simulink model "MdXX_Status"  (R2018b)
settings: Solver=FixedStepDiscrete  StartTime=0.0  StopTime=10.0  FixedStep=0.01  RelTol=1e-3
undefined symbols (not defined in the file or in its folder): data, NvStMdxxMemStatusKam_Set
libraries: RspLib x94, simulink x1
(part 1 of 2)
settings Model: Creator=sn2xws  LastModifiedBy=sn55gm
settings Model: ModifiedHistory=|
  | 25.2.19 V3.8.0 557 上到位置信号的退出，改为不再看是否有不共存的模式启动
  | 25.7.4 V3.13.0 新增Md61 Md62
settings DataIOCC: SaveFormat=StructureWithTime
settings OptimizationCC: DefaultParameterBehavior=Inlined  EnhancedBackFolding=on  PassReuseOutputArgsAs=Individual arguments  ZeroExternalMemoryAtStartup=off  ZeroInternalMemoryAtStartup=off  OptimizeBlockOrder=speed  DifferentSizesBufferReuse=on  OptimizationCustomize=off
settings DebuggingCC: ParameterTunabilityLossMsg=error
settings ModelReferenceCC: ModelReferenceNumInstancesAllowed=Single
settings SFSimCC: MATLABDynamicMemAlloc=off
settings RTWCC: SystemTargetFile=autosar.tlc  GenCodeOnly=on  TemplateMakefile=ert_default_tmf  Description=AUTOSAR  GenerateReport=on  IncludeHyperlinkInReport=on  LaunchReport=on  GenerateTraceInfo=on  GenerateTraceReport=on  GenerateTraceReportSl=on  GenerateTraceReportSf=on  GenerateTraceReportEml=on  GenerateCodeMetricsReport=on
settings CodeAppCC: ForceParamTrailComments=on  IgnoreCustomStorageClasses=off  OperatorAnnotations=on  SimulinkDataObjDesc=on  SFDataObjDesc=on  InsertBlockDesc=on
settings STFCustomTargetCC: TargetLangStandard=C99 (ISO)  MultiwordLength=256  ParMdlRefBuildCompliant=on  CompOptLevelCompliant=on  IncludeMdlTerminateFcn=off  CombineOutputUpdateFcns=on  SuppressErrorStatus=on  ERTCustomFileBanners=on  SupportNonFinite=off  SupportComplex=off  SupportContinuousTime=off  SupportNonInlinedSFcns=off  RemoveResetFunc=on  MATLABClassNameForMDSCustomization=Simulink.SoftwareTarget.ERTCustomization  AutosarCompliant=on  UseToolchainInfoCompliant=on  LookupTableObjectStructAxisOrder=2,1,3,4,...  LUTObjectStructOrderEvenSpacing=Size,Table,Breakpoints  SystemTargetFile=autosar.tlc
settings ERTTargetCC: TargetLangStandard=C99 (ISO)  ConcurrentExecutionCompliant=off  IncludeMdlTerminateFcn=off  SuppressErrorStatus=on  SupportNonFinite=off  SupportComplex=off  ModelStepFunctionPrototypeControlCompliant=off  CPPClassGenCompliant=off  AutosarCompliant=on  LookupTableObjectStructAxisOrder=2,1,3,4,...  LUTObjectStructOrderEvenSpacing=Size,Table,Breakpoints  InlinedParameterPlacement=NonHierarchical  ERTCustomFileTemplate=example_file_process.tlc  ERTFilePackagingFormat=Compact

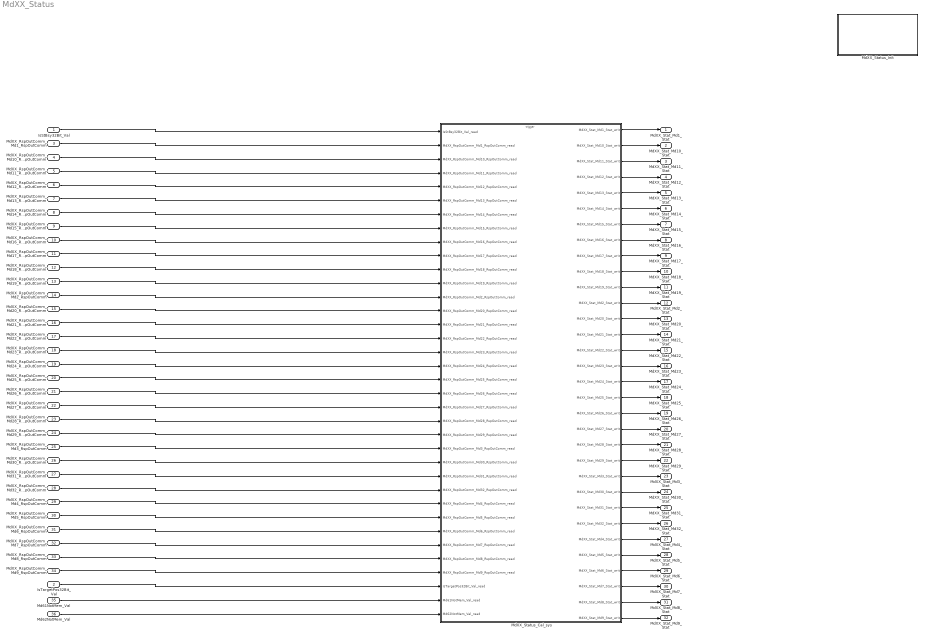
== system MdXX_Status ==
  IsStBsy32Bit_Val : Inport  OutDataTypeStr=uint32  PortDimensions=1
  IsTargetPos32Bit_Val : Inport  Port=2  OutDataTypeStr=uint32  PortDimensions=1
  MdXX_RspOutComm_Md1_RspOutComm : Inport  Port=3  OutDataTypeStr=uint8  PortDimensions=1
  MdXX_RspOutComm_Md10_RspOutComm : Inport  Port=4  OutDataTypeStr=uint8  PortDimensions=1
  MdXX_RspOutComm_Md11_RspOutComm : Inport  Port=5  OutDataTypeStr=uint8  PortDimensions=1
  MdXX_RspOutComm_Md12_RspOutComm : Inport  Port=6  OutDataTypeStr=uint8  PortDimensions=1
  MdXX_RspOutComm_Md13_RspOutComm : Inport  Port=7  OutDataTypeStr=uint8  PortDimensions=1
  MdXX_RspOutComm_Md14_RspOutComm : Inport  Port=8  OutDataTypeStr=uint8  PortDimensions=1
  MdXX_RspOutComm_Md15_RspOutComm : Inport  Port=9  OutDataTypeStr=uint8  PortDimensions=1
  MdXX_RspOutComm_Md16_RspOutComm : Inport  Port=10  OutDataTypeStr=uint8  PortDimensions=1
  MdXX_RspOutComm_Md17_RspOutComm : Inport  Port=11  OutDataTypeStr=uint8  PortDimensions=1
  MdXX_RspOutComm_Md18_RspOutComm : Inport  Port=12  OutDataTypeStr=uint8  PortDimensions=1
  MdXX_RspOutComm_Md19_RspOutComm : Inport  Port=13  OutDataTypeStr=uint8  PortDimensions=1
  MdXX_RspOutComm_Md2_RspOutComm : Inport  Port=14  OutDataTypeStr=uint8  PortDimensions=1
  MdXX_RspOutComm_Md20_RspOutComm : Inport  Port=15  OutDataTypeStr=uint8  PortDimensions=1
  MdXX_RspOutComm_Md21_RspOutComm : Inport  Port=16  OutDataTypeStr=uint8  PortDimensions=1
  MdXX_RspOutComm_Md22_RspOutComm : Inport  Port=17  OutDataTypeStr=uint8  PortDimensions=1
  MdXX_RspOutComm_Md23_RspOutComm : Inport  Port=18  OutDataTypeStr=uint8  PortDimensions=1
  MdXX_RspOutComm_Md24_RspOutComm : Inport  Port=19  OutDataTypeStr=uint8  PortDimensions=1
  MdXX_RspOutComm_Md25_RspOutComm : Inport  Port=20  OutDataTypeStr=uint8  PortDimensions=1
  MdXX_RspOutComm_Md26_RspOutComm : Inport  Port=21  OutDataTypeStr=uint8  PortDimensions=1
  MdXX_RspOutComm_Md27_RspOutComm : Inport  Port=22  OutDataTypeStr=uint8  PortDimensions=1
  MdXX_RspOutComm_Md28_RspOutComm : Inport  Port=23  OutDataTypeStr=uint8  PortDimensions=1
  MdXX_RspOutComm_Md29_RspOutComm : Inport  Port=24  OutDataTypeStr=uint8  PortDimensions=1
  MdXX_RspOutComm_Md3_RspOutComm : Inport  Port=25  OutDataTypeStr=uint8  PortDimensions=1
  MdXX_RspOutComm_Md30_RspOutComm : Inport  Port=26  OutDataTypeStr=uint8  PortDimensions=1
  MdXX_RspOutComm_Md31_RspOutComm : Inport  Port=27  OutDataTypeStr=uint8  PortDimensions=1
  MdXX_RspOutComm_Md32_RspOutComm : Inport  Port=28  OutDataTypeStr=uint8  PortDimensions=1
  MdXX_RspOutComm_Md4_RspOutComm : Inport  Port=29  OutDataTypeStr=uint8  PortDimensions=1
  MdXX_RspOutComm_Md5_RspOutComm : Inport  Port=30  OutDataTypeStr=uint8  PortDimensions=1
  MdXX_RspOutComm_Md6_RspOutComm : Inport  Port=31  OutDataTypeStr=uint8  PortDimensions=1
  MdXX_RspOutComm_Md7_RspOutComm : Inport  Port=32  OutDataTypeStr=uint8  PortDimensions=1
  MdXX_RspOutComm_Md8_RspOutComm : Inport  Port=33  OutDataTypeStr=uint8  PortDimensions=1
  MdXX_RspOutComm_Md9_RspOutComm : Inport  Port=34  OutDataTypeStr=uint8  PortDimensions=1
  Md61NotMem_Val : Inport  Port=35  OutDataTypeStr=boolean  PortDimensions=1
  Md62NotMem_Val : Inport  Port=36  OutDataTypeStr=boolean  PortDimensions=1
  MdXX_Status_Cal_sys : Subsystem
  MdXX_Status_Init : Subsystem
  MdXX_Stat_Md1_Stat : Outport  OutDataTypeStr=uint8  PortDimensions=1
  MdXX_Stat_Md10_Stat : Outport  Port=2  OutDataTypeStr=uint8  PortDimensions=1
  MdXX_Stat_Md11_Stat : Outport  Port=3  OutDataTypeStr=uint8  PortDimensions=1
  MdXX_Stat_Md12_Stat : Outport  Port=4  OutDataTypeStr=uint8  PortDimensions=1
  MdXX_Stat_Md13_Stat : Outport  Port=5  OutDataTypeStr=uint8  PortDimensions=1
  MdXX_Stat_Md14_Stat : Outport  Port=6  OutDataTypeStr=uint8  PortDimensions=1
  MdXX_Stat_Md15_Stat : Outport  Port=7  OutDataTypeStr=uint8  PortDimensions=1
  MdXX_Stat_Md16_Stat : Outport  Port=8  OutDataTypeStr=uint8  PortDimensions=1
  MdXX_Stat_Md17_Stat : Outport  Port=9  OutDataTypeStr=uint8  PortDimensions=1
  MdXX_Stat_Md18_Stat : Outport  Port=10  OutDataTypeStr=uint8  PortDimensions=1
  MdXX_Stat_Md19_Stat : Outport  Port=11  OutDataTypeStr=uint8  PortDimensions=1
  MdXX_Stat_Md2_Stat : Outport  Port=12  OutDataTypeStr=uint8  PortDimensions=1
  MdXX_Stat_Md20_Stat : Outport  Port=13  OutDataTypeStr=uint8  PortDimensions=1
  MdXX_Stat_Md21_Stat : Outport  Port=14  OutDataTypeStr=uint8  PortDimensions=1
  MdXX_Stat_Md22_Stat : Outport  Port=15  OutDataTypeStr=uint8  PortDimensions=1
  MdXX_Stat_Md23_Stat : Outport  Port=16  OutDataTypeStr=uint8  PortDimensions=1
  MdXX_Stat_Md24_Stat : Outport  Port=17  OutDataTypeStr=uint8  PortDimensions=1
  MdXX_Stat_Md25_Stat : Outport  Port=18  OutDataTypeStr=uint8  PortDimensions=1
  MdXX_Stat_Md26_Stat : Outport  Port=19  OutDataTypeStr=uint8  PortDimensions=1
  MdXX_Stat_Md27_Stat : Outport  Port=20  OutDataTypeStr=uint8  PortDimensions=1
  MdXX_Stat_Md28_Stat : Outport  Port=21  OutDataTypeStr=uint8  PortDimensions=1
  MdXX_Stat_Md29_Stat : Outport  Port=22  OutDataTypeStr=uint8  PortDimensions=1
  MdXX_Stat_Md3_Stat : Outport  Port=23  OutDataTypeStr=uint8  PortDimensions=1
  MdXX_Stat_Md30_Stat : Outport  Port=24  OutDataTypeStr=uint8  PortDimensions=1
  MdXX_Stat_Md31_Stat : Outport  Port=25  OutDataTypeStr=uint8  PortDimensions=1
  MdXX_Stat_Md32_Stat : Outport  Port=26  OutDataTypeStr=uint8  PortDimensions=1
  MdXX_Stat_Md4_Stat : Outport  Port=27  OutDataTypeStr=uint8  PortDimensions=1
  MdXX_Stat_Md5_Stat : Outport  Port=28  OutDataTypeStr=uint8  PortDimensions=1
  MdXX_Stat_Md6_Stat : Outport  Port=29  OutDataTypeStr=uint8  PortDimensions=1
  MdXX_Stat_Md7_Stat : Outport  Port=30  OutDataTypeStr=uint8  PortDimensions=1
  MdXX_Stat_Md8_Stat : Outport  Port=31  OutDataTypeStr=uint8  PortDimensions=1
  MdXX_Stat_Md9_Stat : Outport  Port=32  OutDataTypeStr=uint8  PortDimensions=1
  wires:
  IsStBsy32Bit_Val/1 -> MdXX_Status_Cal_sys/1(IsStBsy32Bit_Val_read)
  IsTargetPos32Bit_Val/1 -> MdXX_Status_Cal_sys/34(IsTargetPos32Bit_Val_read)
  MdXX_RspOutComm_Md1_RspOutComm/1 -> MdXX_Status_Cal_sys/2(MdXX_RspOutComm_Md1_RspOutComm_read)
  MdXX_RspOutComm_Md10_RspOutComm/1 -> MdXX_Status_Cal_sys/3(MdXX_RspOutComm_Md10_RspOutComm_read)
  MdXX_RspOutComm_Md11_RspOutComm/1 -> MdXX_Status_Cal_sys/4(MdXX_RspOutComm_Md11_RspOutComm_read)
  MdXX_RspOutComm_Md12_RspOutComm/1 -> MdXX_Status_Cal_sys/5(MdXX_RspOutComm_Md12_RspOutComm_read)
  MdXX_RspOutComm_Md13_RspOutComm/1 -> MdXX_Status_Cal_sys/6(MdXX_RspOutComm_Md13_RspOutComm_read)
  MdXX_RspOutComm_Md14_RspOutComm/1 -> MdXX_Status_Cal_sys/7(MdXX_RspOutComm_Md14_RspOutComm_read)
  MdXX_RspOutComm_Md15_RspOutComm/1 -> MdXX_Status_Cal_sys/8(MdXX_RspOutComm_Md15_RspOutComm_read)
  MdXX_RspOutComm_Md16_RspOutComm/1 -> MdXX_Status_Cal_sys/9(MdXX_RspOutComm_Md16_RspOutComm_read)
  MdXX_RspOutComm_Md17_RspOutComm/1 -> MdXX_Status_Cal_sys/10(MdXX_RspOutComm_Md17_RspOutComm_read)
  MdXX_RspOutComm_Md18_RspOutComm/1 -> MdXX_Status_Cal_sys/11(MdXX_RspOutComm_Md18_RspOutComm_read)
  MdXX_RspOutComm_Md19_RspOutComm/1 -> MdXX_Status_Cal_sys/12(MdXX_RspOutComm_Md19_RspOutComm_read)
  MdXX_RspOutComm_Md2_RspOutComm/1 -> MdXX_Status_Cal_sys/13(MdXX_RspOutComm_Md2_RspOutComm_read)
  MdXX_RspOutComm_Md20_RspOutComm/1 -> MdXX_Status_Cal_sys/14(MdXX_RspOutComm_Md20_RspOutComm_read)
  MdXX_RspOutComm_Md21_RspOutComm/1 -> MdXX_Status_Cal_sys/15(MdXX_RspOutComm_Md21_RspOutComm_read)
  MdXX_RspOutComm_Md22_RspOutComm/1 -> MdXX_Status_Cal_sys/16(MdXX_RspOutComm_Md22_RspOutComm_read)
  MdXX_RspOutComm_Md23_RspOutComm/1 -> MdXX_Status_Cal_sys/17(MdXX_RspOutComm_Md23_RspOutComm_read)
  MdXX_RspOutComm_Md24_RspOutComm/1 -> MdXX_Status_Cal_sys/18(MdXX_RspOutComm_Md24_RspOutComm_read)
  MdXX_RspOutComm_Md25_RspOutComm/1 -> MdXX_Status_Cal_sys/19(MdXX_RspOutComm_Md25_RspOutComm_read)
  MdXX_RspOutComm_Md26_RspOutComm/1 -> MdXX_Status_Cal_sys/20(MdXX_RspOutComm_Md26_RspOutComm_read)
  MdXX_RspOutComm_Md27_RspOutComm/1 -> MdXX_Status_Cal_sys/21(MdXX_RspOutComm_Md27_RspOutComm_read)
  MdXX_RspOutComm_Md28_RspOutComm/1 -> MdXX_Status_Cal_sys/22(MdXX_RspOutComm_Md28_RspOutComm_read)
  MdXX_RspOutComm_Md29_RspOutComm/1 -> MdXX_Status_Cal_sys/23(MdXX_RspOutComm_Md29_RspOutComm_read)
  MdXX_RspOutComm_Md3_RspOutComm/1 -> MdXX_Status_Cal_sys/24(MdXX_RspOutComm_Md3_RspOutComm_read)
  MdXX_RspOutComm_Md30_RspOutComm/1 -> MdXX_Status_Cal_sys/25(MdXX_RspOutComm_Md30_RspOutComm_read)
  MdXX_RspOutComm_Md31_RspOutComm/1 -> MdXX_Status_Cal_sys/26(MdXX_RspOutComm_Md31_RspOutComm_read)
  MdXX_RspOutComm_Md32_RspOutComm/1 -> MdXX_Status_Cal_sys/27(MdXX_RspOutComm_Md32_RspOutComm_read)
  MdXX_RspOutComm_Md4_RspOutComm/1 -> MdXX_Status_Cal_sys/28(MdXX_RspOutComm_Md4_RspOutComm_read)
  MdXX_RspOutComm_Md5_RspOutComm/1 -> MdXX_Status_Cal_sys/29(MdXX_RspOutComm_Md5_RspOutComm_read)
  MdXX_RspOutComm_Md6_RspOutComm/1 -> MdXX_Status_Cal_sys/30(MdXX_RspOutComm_Md6_RspOutComm_read)
  MdXX_RspOutComm_Md7_RspOutComm/1 -> MdXX_Status_Cal_sys/31(MdXX_RspOutComm_Md7_RspOutComm_read)
  MdXX_RspOutComm_Md8_RspOutComm/1 -> MdXX_Status_Cal_sys/32(MdXX_RspOutComm_Md8_RspOutComm_read)
  MdXX_RspOutComm_Md9_RspOutComm/1 -> MdXX_Status_Cal_sys/33(MdXX_RspOutComm_Md9_RspOutComm_read)
  MdXX_Status_Cal_sys/1(MdXX_Stat_Md1_Stat_write) -> MdXX_Stat_Md1_Stat/1
  MdXX_Status_Cal_sys/2(MdXX_Stat_Md10_Stat_write) -> MdXX_Stat_Md10_Stat/1
  MdXX_Status_Cal_sys/3(MdXX_Stat_Md11_Stat_write) -> MdXX_Stat_Md11_Stat/1
  MdXX_Status_Cal_sys/4(MdXX_Stat_Md12_Stat_write) -> MdXX_Stat_Md12_Stat/1
  MdXX_Status_Cal_sys/5(MdXX_Stat_Md13_Stat_write) -> MdXX_Stat_Md13_Stat/1
  MdXX_Status_Cal_sys/6(MdXX_Stat_Md14_Stat_write) -> MdXX_Stat_Md14_Stat/1
  MdXX_Status_Cal_sys/7(MdXX_Stat_Md15_Stat_write) -> MdXX_Stat_Md15_Stat/1
  MdXX_Status_Cal_sys/8(MdXX_Stat_Md16_Stat_write) -> MdXX_Stat_Md16_Stat/1
  MdXX_Status_Cal_sys/9(MdXX_Stat_Md17_Stat_write) -> MdXX_Stat_Md17_Stat/1
  MdXX_Status_Cal_sys/10(MdXX_Stat_Md18_Stat_write) -> MdXX_Stat_Md18_Stat/1
  MdXX_Status_Cal_sys/11(MdXX_Stat_Md19_Stat_write) -> MdXX_Stat_Md19_Stat/1
  MdXX_Status_Cal_sys/12(MdXX_Stat_Md2_Stat_write) -> MdXX_Stat_Md2_Stat/1
  MdXX_Status_Cal_sys/13(MdXX_Stat_Md20_Stat_write) -> MdXX_Stat_Md20_Stat/1
  MdXX_Status_Cal_sys/14(MdXX_Stat_Md21_Stat_write) -> MdXX_Stat_Md21_Stat/1
  MdXX_Status_Cal_sys/15(MdXX_Stat_Md22_Stat_write) -> MdXX_Stat_Md22_Stat/1
  MdXX_Status_Cal_sys/16(MdXX_Stat_Md23_Stat_write) -> MdXX_Stat_Md23_Stat/1
  MdXX_Status_Cal_sys/17(MdXX_Stat_Md24_Stat_write) -> MdXX_Stat_Md24_Stat/1
  MdXX_Status_Cal_sys/18(MdXX_Stat_Md25_Stat_write) -> MdXX_Stat_Md25_Stat/1
  MdXX_Status_Cal_sys/19(MdXX_Stat_Md26_Stat_write) -> MdXX_Stat_Md26_Stat/1
  MdXX_Status_Cal_sys/20(MdXX_Stat_Md27_Stat_write) -> MdXX_Stat_Md27_Stat/1
  MdXX_Status_Cal_sys/21(MdXX_Stat_Md28_Stat_write) -> MdXX_Stat_Md28_Stat/1
  MdXX_Status_Cal_sys/22(MdXX_Stat_Md29_Stat_write) -> MdXX_Stat_Md29_Stat/1
  MdXX_Status_Cal_sys/23(MdXX_Stat_Md3_Stat_write) -> MdXX_Stat_Md3_Stat/1
  MdXX_Status_Cal_sys/24(MdXX_Stat_Md30_Stat_write) -> MdXX_Stat_Md30_Stat/1
  MdXX_Status_Cal_sys/25(MdXX_Stat_Md31_Stat_write) -> MdXX_Stat_Md31_Stat/1
  MdXX_Status_Cal_sys/26(MdXX_Stat_Md32_Stat_write) -> MdXX_Stat_Md32_Stat/1
  MdXX_Status_Cal_sys/27(MdXX_Stat_Md4_Stat_write) -> MdXX_Stat_Md4_Stat/1
  MdXX_Status_Cal_sys/28(MdXX_Stat_Md5_Stat_write) -> MdXX_Stat_Md5_Stat/1
  MdXX_Status_Cal_sys/29(MdXX_Stat_Md6_Stat_write) -> MdXX_Stat_Md6_Stat/1
  MdXX_Status_Cal_sys/30(MdXX_Stat_Md7_Stat_write) -> MdXX_Stat_Md7_Stat/1
  MdXX_Status_Cal_sys/31(MdXX_Stat_Md8_Stat_write) -> MdXX_Stat_Md8_Stat/1
  MdXX_Status_Cal_sys/32(MdXX_Stat_Md9_Stat_write) -> MdXX_Stat_Md9_Stat/1
  Md61NotMem_Val/1 -> MdXX_Status_Cal_sys/35(Md61NotMem_Val_read)
  Md62NotMem_Val/1 -> MdXX_Status_Cal_sys/36(Md62NotMem_Val_read)

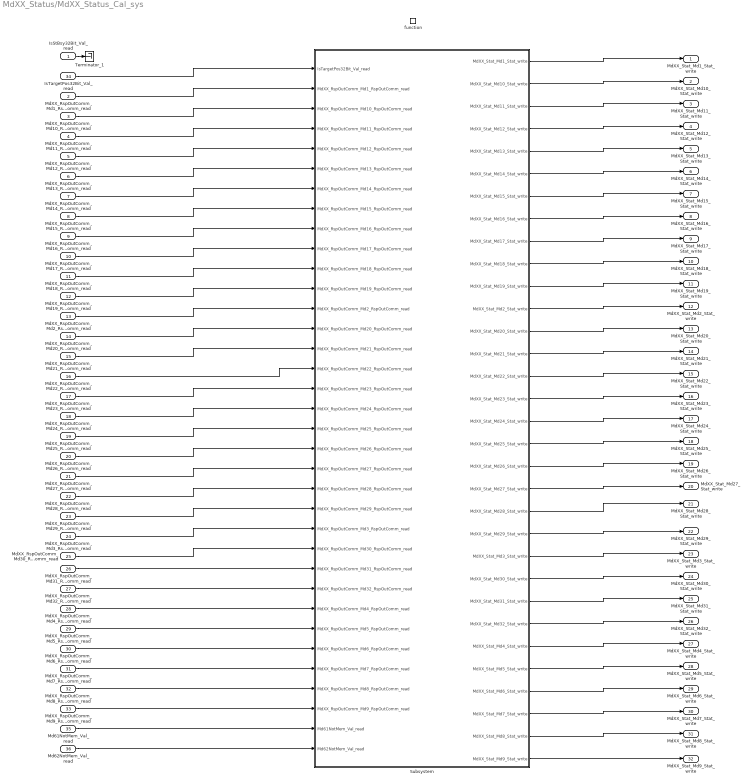
== system MdXX_Status/MdXX_Status_Cal_sys ==
  IsStBsy32Bit_Val_read : Inport
  MdXX_RspOutComm_Md1_RspOutComm_read : Inport  Port=2
  MdXX_RspOutComm_Md10_RspOutComm_read : Inport  Port=3
  MdXX_RspOutComm_Md11_RspOutComm_read : Inport  Port=4
  MdXX_RspOutComm_Md12_RspOutComm_read : Inport  Port=5
  MdXX_RspOutComm_Md13_RspOutComm_read : Inport  Port=6
  MdXX_RspOutComm_Md14_RspOutComm_read : Inport  Port=7
  MdXX_RspOutComm_Md15_RspOutComm_read : Inport  Port=8
  MdXX_RspOutComm_Md16_RspOutComm_read : Inport  Port=9
  MdXX_RspOutComm_Md17_RspOutComm_read : Inport  Port=10
  MdXX_RspOutComm_Md18_RspOutComm_read : Inport  Port=11
  MdXX_RspOutComm_Md19_RspOutComm_read : Inport  Port=12
  MdXX_RspOutComm_Md2_RspOutComm_read : Inport  Port=13
  MdXX_RspOutComm_Md20_RspOutComm_read : Inport  Port=14
  MdXX_RspOutComm_Md21_RspOutComm_read : Inport  Port=15
  MdXX_RspOutComm_Md22_RspOutComm_read : Inport  Port=16
  MdXX_RspOutComm_Md23_RspOutComm_read : Inport  Port=17
  MdXX_RspOutComm_Md24_RspOutComm_read : Inport  Port=18
  MdXX_RspOutComm_Md25_RspOutComm_read : Inport  Port=19
  MdXX_RspOutComm_Md26_RspOutComm_read : Inport  Port=20
  MdXX_RspOutComm_Md27_RspOutComm_read : Inport  Port=21
  MdXX_RspOutComm_Md28_RspOutComm_read : Inport  Port=22
  MdXX_RspOutComm_Md29_RspOutComm_read : Inport  Port=23
  MdXX_RspOutComm_Md3_RspOutComm_read : Inport  Port=24
  MdXX_RspOutComm_Md30_RspOutComm_read : Inport  Port=25
  MdXX_RspOutComm_Md31_RspOutComm_read : Inport  Port=26
  MdXX_RspOutComm_Md32_RspOutComm_read : Inport  Port=27
  MdXX_RspOutComm_Md4_RspOutComm_read : Inport  Port=28
  MdXX_RspOutComm_Md5_RspOutComm_read : Inport  Port=29
  MdXX_RspOutComm_Md6_RspOutComm_read : Inport  Port=30
  MdXX_RspOutComm_Md7_RspOutComm_read : Inport  Port=31
  MdXX_RspOutComm_Md8_RspOutComm_read : Inport  Port=32
  MdXX_RspOutComm_Md9_RspOutComm_read : Inport  Port=33
  IsTargetPos32Bit_Val_read : Inport  Port=34
  Md61NotMem_Val_read : Inport  Port=35
  Md62NotMem_Val_read : Inport  Port=36
  function : TriggerPort  TriggerType=function-call  IsSimulinkFunction=on  FunctionName=MdXX_Status_Cal  VariantControl=(inherit)
  Subsystem : Subsystem
  Terminator_1 : Terminator
  MdXX_Stat_Md1_Stat_write : Outport  InitialOutput=0
  MdXX_Stat_Md10_Stat_write : Outport  Port=2  InitialOutput=0
  MdXX_Stat_Md11_Stat_write : Outport  Port=3  InitialOutput=0
  MdXX_Stat_Md12_Stat_write : Outport  Port=4  InitialOutput=0
  MdXX_Stat_Md13_Stat_write : Outport  Port=5  InitialOutput=0
  MdXX_Stat_Md14_Stat_write : Outport  Port=6  InitialOutput=0
  MdXX_Stat_Md15_Stat_write : Outport  Port=7  InitialOutput=0
  MdXX_Stat_Md16_Stat_write : Outport  Port=8  InitialOutput=0
  MdXX_Stat_Md17_Stat_write : Outport  Port=9  InitialOutput=0
  MdXX_Stat_Md18_Stat_write : Outport  Port=10  InitialOutput=0
  MdXX_Stat_Md19_Stat_write : Outport  Port=11  InitialOutput=0
  MdXX_Stat_Md2_Stat_write : Outport  Port=12  InitialOutput=0
  MdXX_Stat_Md20_Stat_write : Outport  Port=13  InitialOutput=0
  MdXX_Stat_Md21_Stat_write : Outport  Port=14  InitialOutput=0
  MdXX_Stat_Md22_Stat_write : Outport  Port=15  InitialOutput=0
  MdXX_Stat_Md23_Stat_write : Outport  Port=16  InitialOutput=0
  MdXX_Stat_Md24_Stat_write : Outport  Port=17  InitialOutput=0
  MdXX_Stat_Md25_Stat_write : Outport  Port=18  InitialOutput=0
  MdXX_Stat_Md26_Stat_write : Outport  Port=19  InitialOutput=0
  MdXX_Stat_Md27_Stat_write : Outport  Port=20  InitialOutput=0
  MdXX_Stat_Md28_Stat_write : Outport  Port=21  InitialOutput=0
  MdXX_Stat_Md29_Stat_write : Outport  Port=22  InitialOutput=0
  MdXX_Stat_Md3_Stat_write : Outport  Port=23  InitialOutput=0
  MdXX_Stat_Md30_Stat_write : Outport  Port=24  InitialOutput=0
  MdXX_Stat_Md31_Stat_write : Outport  Port=25  InitialOutput=0
  MdXX_Stat_Md32_Stat_write : Outport  Port=26  InitialOutput=0
  MdXX_Stat_Md4_Stat_write : Outport  Port=27  InitialOutput=0
  MdXX_Stat_Md5_Stat_write : Outport  Port=28  InitialOutput=0
  MdXX_Stat_Md6_Stat_write : Outport  Port=29  InitialOutput=0
  MdXX_Stat_Md7_Stat_write : Outport  Port=30  InitialOutput=0
  MdXX_Stat_Md8_Stat_write : Outport  Port=31  InitialOutput=0
  MdXX_Stat_Md9_Stat_write : Outport  Port=32  InitialOutput=0
  wires:
  Subsystem/1(MdXX_Stat_Md1_Stat_write) -> MdXX_Stat_Md1_Stat_write/1
  Subsystem/2(MdXX_Stat_Md10_Stat_write) -> MdXX_Stat_Md10_Stat_write/1
  Subsystem/3(MdXX_Stat_Md11_Stat_write) -> MdXX_Stat_Md11_Stat_write/1
  Subsystem/4(MdXX_Stat_Md12_Stat_write) -> MdXX_Stat_Md12_Stat_write/1
  Subsystem/5(MdXX_Stat_Md13_Stat_write) -> MdXX_Stat_Md13_Stat_write/1
  Subsystem/6(MdXX_Stat_Md14_Stat_write) -> MdXX_Stat_Md14_Stat_write/1
  Subsystem/7(MdXX_Stat_Md15_Stat_write) -> MdXX_Stat_Md15_Stat_write/1
  Subsystem/8(MdXX_Stat_Md16_Stat_write) -> MdXX_Stat_Md16_Stat_write/1
  Subsystem/9(MdXX_Stat_Md17_Stat_write) -> MdXX_Stat_Md17_Stat_write/1
  Subsystem/10(MdXX_Stat_Md18_Stat_write) -> MdXX_Stat_Md18_Stat_write/1
  Subsystem/11(MdXX_Stat_Md19_Stat_write) -> MdXX_Stat_Md19_Stat_write/1
  Subsystem/12(MdXX_Stat_Md2_Stat_write) -> MdXX_Stat_Md2_Stat_write/1
  Subsystem/13(MdXX_Stat_Md20_Stat_write) -> MdXX_Stat_Md20_Stat_write/1
  Subsystem/14(MdXX_Stat_Md21_Stat_write) -> MdXX_Stat_Md21_Stat_write/1
  Subsystem/15(MdXX_Stat_Md22_Stat_write) -> MdXX_Stat_Md22_Stat_write/1
  Subsystem/16(MdXX_Stat_Md23_Stat_write) -> MdXX_Stat_Md23_Stat_write/1
  Subsystem/17(MdXX_Stat_Md24_Stat_write) -> MdXX_Stat_Md24_Stat_write/1
  Subsystem/18(MdXX_Stat_Md25_Stat_write) -> MdXX_Stat_Md25_Stat_write/1
  Subsystem/19(MdXX_Stat_Md26_Stat_write) -> MdXX_Stat_Md26_Stat_write/1
  Subsystem/20(MdXX_Stat_Md27_Stat_write) -> MdXX_Stat_Md27_Stat_write/1
  Subsystem/21(MdXX_Stat_Md28_Stat_write) -> MdXX_Stat_Md28_Stat_write/1
  Subsystem/22(MdXX_Stat_Md29_Stat_write) -> MdXX_Stat_Md29_Stat_write/1
  Subsystem/23(MdXX_Stat_Md3_Stat_write) -> MdXX_Stat_Md3_Stat_write/1
  Subsystem/24(MdXX_Stat_Md30_Stat_write) -> MdXX_Stat_Md30_Stat_write/1
  Subsystem/25(MdXX_Stat_Md31_Stat_write) -> MdXX_Stat_Md31_Stat_write/1
  Subsystem/26(MdXX_Stat_Md32_Stat_write) -> MdXX_Stat_Md32_Stat_write/1
  Subsystem/27(MdXX_Stat_Md4_Stat_write) -> MdXX_Stat_Md4_Stat_write/1
  Subsystem/28(MdXX_Stat_Md5_Stat_write) -> MdXX_Stat_Md5_Stat_write/1
  Subsystem/29(MdXX_Stat_Md6_Stat_write) -> MdXX_Stat_Md6_Stat_write/1
  Subsystem/30(MdXX_Stat_Md7_Stat_write) -> MdXX_Stat_Md7_Stat_write/1
  Subsystem/31(MdXX_Stat_Md8_Stat_write) -> MdXX_Stat_Md8_Stat_write/1
  Subsystem/32(MdXX_Stat_Md9_Stat_write) -> MdXX_Stat_Md9_Stat_write/1
  IsTargetPos32Bit_Val_read/1 -> Subsystem/1(IsTargetPos32Bit_Val_read)
  MdXX_RspOutComm_Md1_RspOutComm_read/1 -> Subsystem/2(MdXX_RspOutComm_Md1_RspOutComm_read)
  MdXX_RspOutComm_Md10_RspOutComm_read/1 -> Subsystem/3(MdXX_RspOutComm_Md10_RspOutComm_read)
  MdXX_RspOutComm_Md11_RspOutComm_read/1 -> Subsystem/4(MdXX_RspOutComm_Md11_RspOutComm_read)
  MdXX_RspOutComm_Md12_RspOutComm_read/1 -> Subsystem/5(MdXX_RspOutComm_Md12_RspOutComm_read)
  MdXX_RspOutComm_Md13_RspOutComm_read/1 -> Subsystem/6(MdXX_RspOutComm_Md13_RspOutComm_read)
  MdXX_RspOutComm_Md14_RspOutComm_read/1 -> Subsystem/7(MdXX_RspOutComm_Md14_RspOutComm_read)
  MdXX_RspOutComm_Md15_RspOutComm_read/1 -> Subsystem/8(MdXX_RspOutComm_Md15_RspOutComm_read)
  MdXX_RspOutComm_Md16_RspOutComm_read/1 -> Subsystem/9(MdXX_RspOutComm_Md16_RspOutComm_read)
  MdXX_RspOutComm_Md17_RspOutComm_read/1 -> Subsystem/10(MdXX_RspOutComm_Md17_RspOutComm_read)
  MdXX_RspOutComm_Md18_RspOutComm_read/1 -> Subsystem/11(MdXX_RspOutComm_Md18_RspOutComm_read)
  MdXX_RspOutComm_Md19_RspOutComm_read/1 -> Subsystem/12(MdXX_RspOutComm_Md19_RspOutComm_read)
  MdXX_RspOutComm_Md2_RspOutComm_read/1 -> Subsystem/13(MdXX_RspOutComm_Md2_RspOutComm_read)
  MdXX_RspOutComm_Md20_RspOutComm_read/1 -> Subsystem/14(MdXX_RspOutComm_Md20_RspOutComm_read)
  MdXX_RspOutComm_Md21_RspOutComm_read/1 -> Subsystem/15(MdXX_RspOutComm_Md21_RspOutComm_read)
  MdXX_RspOutComm_Md22_RspOutComm_read/1 -> Subsystem/16(MdXX_RspOutComm_Md22_RspOutComm_read)
  MdXX_RspOutComm_Md23_RspOutComm_read/1 -> Subsystem/17(MdXX_RspOutComm_Md23_RspOutComm_read)
  MdXX_RspOutComm_Md24_RspOutComm_read/1 -> Subsystem/18(MdXX_RspOutComm_Md24_RspOutComm_read)
  MdXX_RspOutComm_Md25_RspOutComm_read/1 -> Subsystem/19(MdXX_RspOutComm_Md25_RspOutComm_read)
  MdXX_RspOutComm_Md26_RspOutComm_read/1 -> Subsystem/20(MdXX_RspOutComm_Md26_RspOutComm_read)
  MdXX_RspOutComm_Md27_RspOutComm_read/1 -> Subsystem/21(MdXX_RspOutComm_Md27_RspOutComm_read)
  MdXX_RspOutComm_Md28_RspOutComm_read/1 -> Subsystem/22(MdXX_RspOutComm_Md28_RspOutComm_read)
  MdXX_RspOutComm_Md29_RspOutComm_read/1 -> Subsystem/23(MdXX_RspOutComm_Md29_RspOutComm_read)
  MdXX_RspOutComm_Md3_RspOutComm_read/1 -> Subsystem/24(MdXX_RspOutComm_Md3_RspOutComm_read)
  MdXX_RspOutComm_Md30_RspOutComm_read/1 -> Subsystem/25(MdXX_RspOutComm_Md30_RspOutComm_read)
  MdXX_RspOutComm_Md31_RspOutComm_read/1 -> Subsystem/26(MdXX_RspOutComm_Md31_RspOutComm_read)
  MdXX_RspOutComm_Md32_RspOutComm_read/1 -> Subsystem/27(MdXX_RspOutComm_Md32_RspOutComm_read)
  MdXX_RspOutComm_Md4_RspOutComm_read/1 -> Subsystem/28(MdXX_RspOutComm_Md4_RspOutComm_read)
  MdXX_RspOutComm_Md5_RspOutComm_read/1 -> Subsystem/29(MdXX_RspOutComm_Md5_RspOutComm_read)
  MdXX_RspOutComm_Md6_RspOutComm_read/1 -> Subsystem/30(MdXX_RspOutComm_Md6_RspOutComm_read)
  MdXX_RspOutComm_Md7_RspOutComm_read/1 -> Subsystem/31(MdXX_RspOutComm_Md7_RspOutComm_read)
  MdXX_RspOutComm_Md8_RspOutComm_read/1 -> Subsystem/32(MdXX_RspOutComm_Md8_RspOutComm_read)
  MdXX_RspOutComm_Md9_RspOutComm_read/1 -> Subsystem/33(MdXX_RspOutComm_Md9_RspOutComm_read)
  Md61NotMem_Val_read/1 -> Subsystem/34(Md61NotMem_Val_read)
  Md62NotMem_Val_read/1 -> Subsystem/35(Md62NotMem_Val_read)
  IsStBsy32Bit_Val_read/1 -> Terminator_1/1

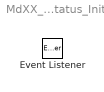
== system MdXX_Status/MdXX_Status_Init ==
  Event Listener : EventListener  EventName=reset
